simulink model "Tester_Controller_A"  (R2024b)
settings: Solver=VariableStepAuto  StartTime=0.0  StopTime=inf  RelTol=1e-3
values from neighbouring files (symbols this model uses):
  clegg = 0.55298    [Lookup_Tables_and_Initializer.m]
  D1 = 0.051209    [Lookup_Tables_and_Initializer.m]
  D2 = 0.050783    [Lookup_Tables_and_Initializer.m]
  E_table = E(V_range2,h_funct(Max_Terminal_V_factor),Sharpness_Const)    [Lookup_Tables.m]    (also in Lookup_Tables_and_Initializer.m)
  I1 = 1.3154    [Lookup_Tables_and_Initializer.m]
  I2 = 0.51307    [Lookup_Tables_and_Initializer.m]
  P1 = 2.4635    [Lookup_Tables_and_Initializer.m]
  P2 = 0.29756    [Lookup_Tables_and_Initializer.m]
  V_range2 = 0:0.01:1.44    [Lookup_Tables.m]    (also in Lookup_Tables_and_Initializer.m)
undefined symbols (not defined in the file or in its folder): DiscIntNeverNeededParam
libraries: simulink x3, slpidlib x3, eeGeneralControl x2, instrumentlib x2, dspstat3 x1, dspindex x1, realtime_pacer_lib x1, SignalEditorBlockLib x1
settings Model: Creator=errikos  LastModifiedBy=sh2323
settings SolverCC: AlgebraicLoopSolver=TrustRegion
settings DataIOCC: ReturnWorkspaceOutputs=off
settings DebuggingCC: UnconnectedInputMsg=warning  UnconnectedOutputMsg=warning  UnconnectedLineMsg=warning  ArithmeticOperatorsInVariantConditions=warning
settings ModelReferenceCC: EnableRefExpFcnMdlSchedulingChecks=on
settings SFSimCC: CustomCodeUndefinedFunction=UseInterfaceOnly
settings RTWCC: GPUComputeCapability=3.5  DLArmComputeVersion=19.05

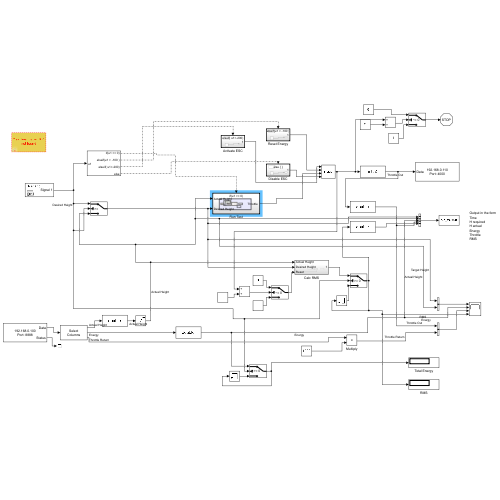
[thumbnail: Simulink's stored preview of the top-level diagram]
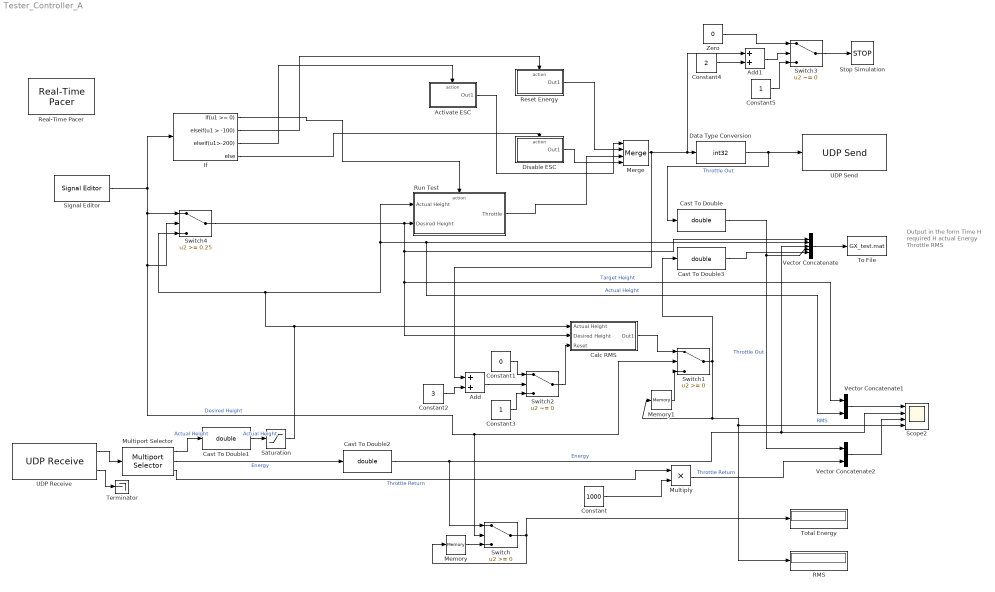
== system Tester_Controller_A ==
  note: Output in the form
      | Time
      | H required
      | H actual
      | Energy
      | Throttle
      | RMS
  Activate ESC : Subsystem  TreatAsAtomicUnit=on
  Add : Sum
  Add1 : Sum
  Calc RMS : Subsystem
  Cast To Double{,1..3} (4 alike) : DataTypeConversion  OutDataTypeStr=double  SaturateOnIntegerOverflow=off  RndMeth=Floor
  Constant : Constant  Value=1000
  Constant1 : Constant  Value=0
  Constant2 : Constant  Value=3
  Constant3 : Constant
  Constant4 : Constant  Value=2
  Constant5 : Constant
  Data Type Conversion : DataTypeConversion  OutDataTypeStr=int32  SaturateOnIntegerOverflow=off  RndMeth=Floor
  Disable ESC : Subsystem  TreatAsAtomicUnit=on
  If : If  IfExpression=u1 >= 0  ElseIfExpressions=u1 > -100 , u1>-200
  Memory : Memory
  Memory1 : Memory
  Merge : Merge  Inputs=4
  Multiply : Product
  Multiport Selector : dspindex/Multiport Selector  rowsOrCols=Columns  idxCellArray={ 1, 2,3}  idxErrMode=Clip and Warn
  RMS : Display
  Real-Time Pacer : realtime_pacer_lib/Real-Time Pacer  simTimePerRealTime=1
  Reset Energy : Subsystem  TreatAsAtomicUnit=on
  Run Test : Subsystem  TreatAsAtomicUnit=on
  Saturation : Saturate  UpperLimit=1.7  LowerLimit=0
  Scope2 : Scope  NumInputPorts=4
  Signal Editor : SignalEditorBlockLib/Signal Editor  FileName=/Users/errikoslevis/Downloads/Simulink Testing/samplemission.mat  ActiveScenario=Scenario  ActiveSignal=Signal 1  IsBus=off  OutputBusObjectStr=Bus: BusObject  SampleTime=0.05  ZeroCross=off  OutputAfterFinalValue=Setting to zero  Unit=inherit  PreserveSignalName=on  ApplySigPropsToAllScenarios=on  ApplySigPropsToAllSignals=off
  Stop Simulation : Stop
  Switch : Switch  SaturateOnIntegerOverflow=off  InputSameDT=off
  Switch1 : Switch  SaturateOnIntegerOverflow=off  InputSameDT=off
  Switch2 : Switch  Criteria=u2 ~= 0  SaturateOnIntegerOverflow=off  InputSameDT=off
  Switch3 : Switch  Criteria=u2 ~= 0  ZeroCross=off  SaturateOnIntegerOverflow=off  InputSameDT=off
  Switch4 : Switch  Threshold=0.25  SaturateOnIntegerOverflow=off  InputSameDT=off
  Terminator : Terminator
  To File : ToFile  Filename=GX_test.mat
  Total Energy : Display
  UDP Receive : instrumentlib/UDP Receive  LocalAddress=192.168.0.100  LocalPort=8888  EnablePortSharing=on  Host=192.168.0.110  Port=4000  GetLatestData=on  DataSize="[1  3]"  DataType=single  ASCIIFormatting=%f%f  Terminator=LF  CustomTerminator=10  ByteOrder=little-endian  EnableBlockingMode=off  Timeout=10  SampleTime=0.05  SimulateUsing=Interpreted execution
  UDP Send : instrumentlib/UDP Send  Host=192.168.0.110  Port=4000  LocalAddress=192.168.0.100  LocalPort=-1  EnablePortSharing=on  OutputDatagramPacketSize=4  ByteOrder=little-endian  EnableBlockingMode=on  SimulateUsing=Interpreted execution
  Vector Concatenate : Concatenate  NumInputs=5
  Vector Concatenate1 : Concatenate
  Vector Concatenate2 : Concatenate
  Zero : Constant  Value=0  OutDataTypeStr=Inherit: Inherit via back propagation
  wires:
  UDP Receive/1 -> Multiport Selector/1
  Multiport Selector/1 -> Cast To Double1/1  "Actual Height"
  Multiport Selector/2 -> Cast To Double2/1  "Energy"
  Run Test/1("Throttle ") -> Merge/3
  Data Type Conversion/1 -> Cast To Double/1, UDP Send/1  "Throttle Out"
  Multiport Selector/3 -> Multiply/1  "Throttle Return"
  Multiply/1 -> Vector Concatenate2/2  "Throttle Return"
  Constant/1 -> Multiply/2
  Signal Editor/1 -> Switch4/2, Switch1/2, Switch/2, Switch4/1, If/1  "Desired Height"
  Merge/1 -> Add/1, Add1/1, Data Type Conversion/1
  Vector Concatenate/1 -> To File/1
  If/1 -> Run Test/Action
  If/2 -> Reset Energy/Action
  If/3 -> Activate ESC/Action
  If/4 -> Disable ESC/Action
  Activate ESC/1(Out1) -> Merge/1
  Disable ESC/1(Out1) -> Merge/4
  Switch/1 -> Memory/1, Total Energy/1
  Cast To Double/1 -> Vector Concatenate2/1, Vector Concatenate/4  "Throttle Out"
  Saturation/1 -> Switch4/3, Run Test/1(Actual Height), Vector Concatenate1/2, Vector Concatenate/2, Calc RMS/1(Actual Height)  "Actual Height"
  Cast To Double2/1 -> Switch/1, Scope2/2, Vector Concatenate/3  "Energy"
  Cast To Double3/1 -> Vector Concatenate/5
  Memory/1 -> Switch/3
  Switch1/1 -> RMS/1, Scope2/4, Memory1/1, Cast To Double3/1  "RMS"
  Memory1/1 -> Switch1/3
  Calc RMS/1(Out1) -> Switch1/1
  Switch2/1 -> Calc RMS/3(Reset)
  Constant1/1 -> Switch2/1
  Constant2/1 -> Add/2
  Add/1 -> Switch2/2
  Constant3/1 -> Switch2/3
  Reset Energy/1(Out1) -> Merge/2
  Switch3/1 -> Stop Simulation/1
  Zero/1 -> Switch3/1
  Add1/1 -> Switch3/2
  Constant4/1 -> Add1/2
  Constant5/1 -> Switch3/3
  Vector Concatenate2/1 -> Scope2/3
  Vector Concatenate1/1 -> Scope2/1
  Switch4/1 -> Vector Concatenate/1, Vector Concatenate1/1, Calc RMS/2(Desired Height), Run Test/2(Desired Height)  "Target Height"
  Cast To Double1/1 -> Saturation/1  "Actual Height"
  UDP Receive/2 -> Terminator/1

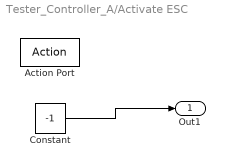
== system Tester_Controller_A/Activate ESC ==
  Action Port : ActionPort  ActionPortLabel=elseif( u1>-200)
  Constant : Constant  Value=-1  SampleTime=0.05
  Out1 : Outport  VectorParamsAs1DForOutWhenUnconnected=off
  wires:
  Constant/1 -> Out1/1

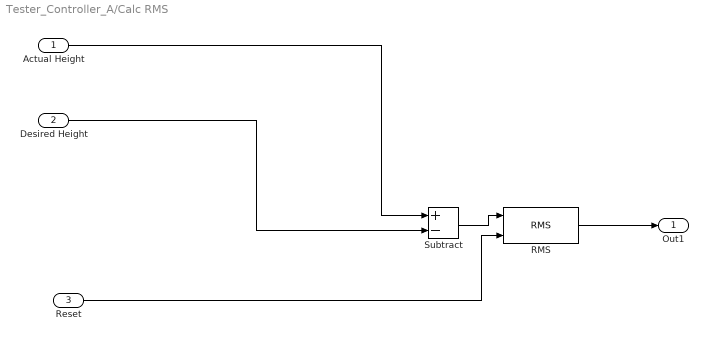
== system Tester_Controller_A/Calc RMS ==
  Actual Height : Inport
  Desired Height : Inport  Port=2
  Reset : Inport  Port=3
  RMS : dspstat3/RMS  run=on  directionMode=Each column  dimension=1  reset_popup=Non-zero sample
  Subtract : Sum  Inputs=+-
  Out1 : Outport  VectorParamsAs1DForOutWhenUnconnected=off
  wires:
  Desired Height/1 -> Subtract/2
  Actual Height/1 -> Subtract/1
  RMS/1 -> Out1/1
  Subtract/1 -> RMS/1
  Reset/1 -> RMS/2

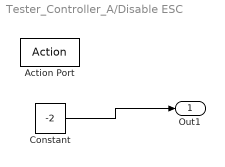
== system Tester_Controller_A/Disable ESC ==
  Action Port : ActionPort  ActionPortLabel=else
  Constant : Constant  Value=-2  SampleTime=0.05
  Out1 : Outport  VectorParamsAs1DForOutWhenUnconnected=off
  wires:
  Constant/1 -> Out1/1

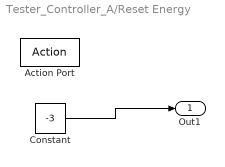
== system Tester_Controller_A/Reset Energy ==
  Action Port : ActionPort  ActionPortLabel=elseif(u1 > -100 )
  Constant : Constant  Value=-3  SampleTime=0.05
  Out1 : Outport  VectorParamsAs1DForOutWhenUnconnected=off
  wires:
  Constant/1 -> Out1/1

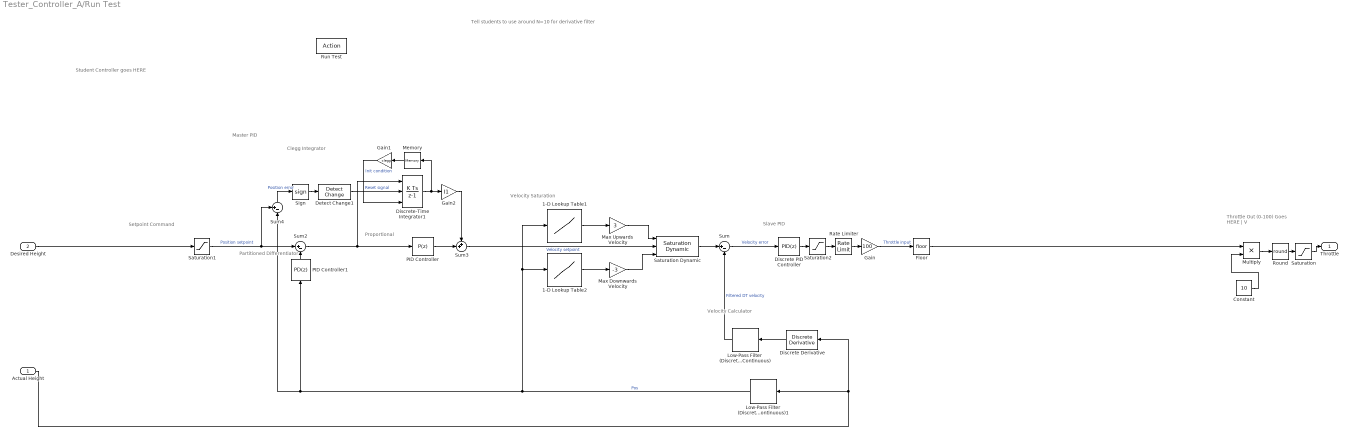
== system Tester_Controller_A/Run Test ==
  note: Tell students to use around N=10 for derivative filter
  note: Throttle Out (0-100)
      | Goes HERE
      |            |
      | 	   V
  note: Student Controller goes HERE
  note: Velocity Calculator
  note: Setpoint Command
  note: Partitioned
      | Differentiator
  note: Proportional
  note: Clegg Integrator
  note: Master
      | PID
  note: Velocity Saturation
  note: Slave PID
  Actual Height : Inport
  Desired Height : Inport  Port=2
  Run Test : ActionPort  ActionPortLabel=if(u1 >= 0)
  1-D Lookup Table1 : Lookup_n-D  NumberOfTableDimensions=1  BreakpointsForDimension1=V_range2  Table=flip(E_table)  InterpMethod=Nearest  InternalRulePriority=Speed  RndMeth=Simplest
  1-D Lookup Table2 : Lookup_n-D  NumberOfTableDimensions=1  BreakpointsForDimension1=V_range2  Table=E_table  InterpMethod=Nearest  InternalRulePriority=Speed  RndMeth=Simplest
  Constant : Constant  Value=10
  Detect Change1 : simulink/Logic and Bit Operations/Detect Change  vinit=0  OutDataTypeStr=boolean
  Discrete Derivative : simulink/Discrete/Discrete Derivative  gainval=1.0  ICPrevScaledInput=0.0  OutMin=[]  OutMax=[]  OutDataType=fixdt(1, 16)  OutScaling=2^-10  DoSatur=off
  Discrete PID Controller : slpidlib/PID Controller  Controller=PID  Form=Parallel  TimeDomain=Discrete-time  UseExternalTs=off  SampleTime=-1  IntegratorMethod=Forward Euler  FilterMethod=Forward Euler  ControllerParametersSource=internal  P=P2  I=I2  UseKiTs=off  D=D2  UseExternalDerivativeSource=off  N=10  UseFilter=on  TunerSelectOption=Transfer Function Based (PID Tuner App)  InitialConditionSource=internal  InitialConditionForIntegrator=0  InitialConditionForFilter=0  DifferentiatorICPrevScaledInput=0  ExternalReset=none  TrackingMode=off  Kt=1  LimitOutput=on  SatLimitsSource=internal  UpperSaturationLimit=1  LowerSaturationLimit=0  LinearizeAsGain=off  AntiWindupMode=none  Kb=1  LimitIntegrator=off  UpperIntegratorSaturationLimit=inf  LowerIntegratorSaturationLimit=-inf  POutMin=[]  POutMax=[]  IOutMin=[]  IOutMax=[]  DOutMin=[]  DOutMax=[]  NOutMin=[]  NOutMax=[]  SumOutMin=[]  SumOutMax=[]  SaturationOutMin=[]  SaturationOutMax=[]  PParamMin=[]  PParamMax=[]  IParamMin=[]  IParamMax=[]  DParamMin=[]  DParamMax=[]  NParamMin=[]  NParamMax=[]  KbParamMin=[]  KbParamMax=[]  KtParamMin=[]  KtParamMax=[]  KbOutMin=[]  KbOutMax=[]  KtOutMin=[]  KtOutMax=[]  IntegratorOutMin=[]  IntegratorOutMax=[]  FilterOutMin=[]  FilterOutMax=[]  SumI1OutMin=[]  SumI1OutMax=[]  SumI2OutMin=[]  SumI2OutMax=[]  SumI3OutMin=[]  SumI3OutMax=[]  SumI4OutMin=[]  SumI4OutMax=[]  SumDOutMin=[]  SumDOutMax=[]  DifferentiatorOutMin=[]  DifferentiatorOutMax=[]  FilterDiffOutCoefMin=[]  FilterDiffOutCoefMax=[]  ReciprocalOutMin=[]  ReciprocalOutMax=[]  SumDenOutMin=[]  SumDenOutMax=[]  SumNumOutMin=[]  SumNumOutMax=[]  DivideOutMin=[]  DivideOutMax=[]  UdiffTsProdOutMin=[]  UdiffTsProdOutMax=[]  NTsProdOutMin=[]  NTsProdOutMax=[]  UintegralTsProdOutMin=[]  UintegralTsProdOutMax=[]  UngainTsProdOutMin=[]  UngainTsProdOutMax=[]  ClampingZeroOutDataTypeStr=Inherit: Inherit via back propagation  ClampingZeroOutMin=[]  ClampingZeroOutMax=[]  FilterDenConstantOutDataTypeStr=Inherit: Inherit via back propagation  FilterDenConstantOutMin=[]  FilterDenConstantOutMax=[]  PCopyOutDataTypeStr=Inherit: Inherit via back propagation  PCopyOutMin=[]  PCopyOutMax=[]  NCopyOutDataTypeStr=Inherit: Inherit via back propagation  NCopyOutMin=[]  NCopyOutMax=[]  IntegratorContinuousStateAttributes=''  IntegratorStateMustResolveToSignalObject=off  IntegratorRTWStateStorageClass=Auto  FilterContinuousStateAttributes=''  FilterStateMustResolveToSignalObject=off  FilterRTWStateStorageClass=Auto  ParallelPVariant=InternalParameters  IdealPVariant=Disabled  IVariant=InternalParameters  DVariant=InternalParameters  IntegratorVariant=Discrete  SatVariant=Enabled  AWVariant=Passthrough  PCopyVariant=Disabled  TRVariant=Disabled  FdbkBlocksVariant=Forward  IdealPFdbkVariant=Disabled  SatFdbkVariant=Disabled  DerivativeFilterVariant=ForwardEulerFilter  NVariant=InternalParameters  NCopyVariant=Disabled  FilterICVariant=InternalICsFilter  IntegratorICVariant=InternalICs  ExternalResetVariant=Disabled  TRSumVariant=Passthrough  SumFdbkVariant=Disabled  SumVariant=Sum_PID  TsampFilterVariant=InternalTs  TsampNgainVariant=Passthrough  TsampIntegralVariant=Disabled_SignalSpec  ExternalSaturationOutDataTypeStr=Inherit: Same as second input  DerivativeSourceVariant=ErrorSignal  PreIntVariant=InternalPreInt
      settings: LibrarySourceBlock=simulink/Discrete/Discrete PID Controller
  Discrete-Time Integrator1 : DiscreteIntegrator  ExternalReset=level  InitialConditionSource=external  SampleTime=-1  ICPrevOutput=DiscIntNeverNeededParam  ICPrevScaledInput=DiscIntNeverNeededParam
  Floor : Rounding
  Gain : Gain  Gain=100
  Gain1 : Gain  Gain=clegg
  Gain2 : Gain  Gain=I1
  Low-Pass Filter (Discrete or Continuous) : eeGeneralControl/Low-Pass Filter (Discrete or Continuous)  K=1  T=0.075  B=inf  A=-inf  init_option=Inherited from block input  x0=0  Ts=-1
  Low-Pass Filter (Discrete or Continuous)1 : eeGeneralControl/Low-Pass Filter (Discrete or Continuous)  K=1  T=0.075  B=inf  A=-inf  init_option=Inherited from block input  x0=0  Ts=-1
  Max Downwards Velocity : Gain  Gain=-3
  Max Upwards Velocity : Gain  Gain=3
  Memory : Memory
  Multiply : Product
  PID Controller : slpidlib/PID Controller  Controller=P  Form=Parallel  TimeDomain=Discrete-time  UseExternalTs=off  SampleTime=-1  IntegratorMethod=Forward Euler  FilterMethod=Forward Euler  ControllerParametersSource=internal  P=P1  I=4  UseKiTs=off  D=0  UseExternalDerivativeSource=off  N=10  UseFilter=on  TunerSelectOption=Transfer Function Based (PID Tuner App)  InitialConditionSource=internal  InitialConditionForIntegrator=0  InitialConditionForFilter=0  DifferentiatorICPrevScaledInput=0  ExternalReset=none  TrackingMode=off  Kt=1  LimitOutput=off  SatLimitsSource=internal  UpperSaturationLimit=inf  LowerSaturationLimit=-inf  LinearizeAsGain=on  AntiWindupMode=none  Kb=1  LimitIntegrator=off  UpperIntegratorSaturationLimit=inf  LowerIntegratorSaturationLimit=-inf  POutMin=[]  POutMax=[]  IOutMin=[]  IOutMax=[]  DOutMin=[]  DOutMax=[]  NOutMin=[]  NOutMax=[]  SumOutMin=[]  SumOutMax=[]  SaturationOutMin=[]  SaturationOutMax=[]  PParamMin=[]  PParamMax=[]  IParamMin=[]  IParamMax=[]  DParamMin=[]  DParamMax=[]  NParamMin=[]  NParamMax=[]  KbParamMin=[]  KbParamMax=[]  KtParamMin=[]  KtParamMax=[]  KbOutMin=[]  KbOutMax=[]  KtOutMin=[]  KtOutMax=[]  IntegratorOutMin=[]  IntegratorOutMax=[]  FilterOutMin=[]  FilterOutMax=[]  SumI1OutMin=[]  SumI1OutMax=[]  SumI2OutMin=[]  SumI2OutMax=[]  SumI3OutMin=[]  SumI3OutMax=[]  SumI4OutMin=[]  SumI4OutMax=[]  SumDOutMin=[]  SumDOutMax=[]  DifferentiatorOutMin=[]  DifferentiatorOutMax=[]  FilterDiffOutCoefMin=[]  FilterDiffOutCoefMax=[]  ReciprocalOutMin=[]  ReciprocalOutMax=[]  SumDenOutMin=[]  SumDenOutMax=[]  SumNumOutMin=[]  SumNumOutMax=[]  DivideOutMin=[]  DivideOutMax=[]  UdiffTsProdOutMin=[]  UdiffTsProdOutMax=[]  NTsProdOutMin=[]  NTsProdOutMax=[]  UintegralTsProdOutMin=[]  UintegralTsProdOutMax=[]  UngainTsProdOutMin=[]  UngainTsProdOutMax=[]  ClampingZeroOutDataTypeStr=Inherit: Inherit via back propagation  ClampingZeroOutMin=[]  ClampingZeroOutMax=[]  FilterDenConstantOutDataTypeStr=Inherit: Inherit via back propagation  FilterDenConstantOutMin=[]  FilterDenConstantOutMax=[]  PCopyOutDataTypeStr=Inherit: Inherit via back propagation  PCopyOutMin=[]  PCopyOutMax=[]  NCopyOutDataTypeStr=Inherit: Inherit via back propagation  NCopyOutMin=[]  NCopyOutMax=[]  IntegratorContinuousStateAttributes=''  IntegratorStateMustResolveToSignalObject=off  IntegratorRTWStateStorageClass=Auto  FilterContinuousStateAttributes=''  FilterStateMustResolveToSignalObject=off  FilterRTWStateStorageClass=Auto  ParallelPVariant=InternalParameters  IdealPVariant=Disabled  IVariant=Disabled  DVariant=Disabled  IntegratorVariant=Disabled  SatVariant=Disabled  AWVariant=Disabled  PCopyVariant=Disabled  TRVariant=Disabled  FdbkBlocksVariant=Forward  IdealPFdbkVariant=Disabled  SatFdbkVariant=Disabled  DerivativeFilterVariant=Disabled  NVariant=Disabled  NCopyVariant=Disabled_SignalSpec  FilterICVariant=Disabled  IntegratorICVariant=Disabled  ExternalResetVariant=Disabled  TRSumVariant=Passthrough  SumFdbkVariant=Disabled  SumVariant=Passthrough_P  TsampFilterVariant=InternalTs  TsampNgainVariant=Passthrough  TsampIntegralVariant=Disabled_SignalSpec  ExternalSaturationOutDataTypeStr=Inherit: Same as second input  DerivativeSourceVariant=Disabled  PreIntVariant=InternalPreInt
  PID Controller1 : slpidlib/PID Controller  Controller=PD  Form=Parallel  TimeDomain=Discrete-time  UseExternalTs=off  SampleTime=-1  IntegratorMethod=Forward Euler  FilterMethod=Forward Euler  ControllerParametersSource=internal  P=1  I=1  UseKiTs=off  D=D1/P1  UseExternalDerivativeSource=off  N=10  UseFilter=on  TunerSelectOption=Transfer Function Based (PID Tuner App)  InitialConditionSource=internal  InitialConditionForIntegrator=0  InitialConditionForFilter=0  DifferentiatorICPrevScaledInput=0  ExternalReset=none  TrackingMode=off  Kt=1  LimitOutput=off  SatLimitsSource=internal  UpperSaturationLimit=inf  LowerSaturationLimit=-inf  LinearizeAsGain=on  AntiWindupMode=none  Kb=1  LimitIntegrator=off  UpperIntegratorSaturationLimit=inf  LowerIntegratorSaturationLimit=-inf  POutMin=[]  POutMax=[]  IOutMin=[]  IOutMax=[]  DOutMin=[]  DOutMax=[]  NOutMin=[]  NOutMax=[]  SumOutMin=[]  SumOutMax=[]  SaturationOutMin=[]  SaturationOutMax=[]  PParamMin=[]  PParamMax=[]  IParamMin=[]  IParamMax=[]  DParamMin=[]  DParamMax=[]  NParamMin=[]  NParamMax=[]  KbParamMin=[]  KbParamMax=[]  KtParamMin=[]  KtParamMax=[]  KbOutMin=[]  KbOutMax=[]  KtOutMin=[]  KtOutMax=[]  IntegratorOutMin=[]  IntegratorOutMax=[]  FilterOutMin=[]  FilterOutMax=[]  SumI1OutMin=[]  SumI1OutMax=[]  SumI2OutMin=[]  SumI2OutMax=[]  SumI3OutMin=[]  SumI3OutMax=[]  SumI4OutMin=[]  SumI4OutMax=[]  SumDOutMin=[]  SumDOutMax=[]  DifferentiatorOutMin=[]  DifferentiatorOutMax=[]  FilterDiffOutCoefMin=[]  FilterDiffOutCoefMax=[]  ReciprocalOutMin=[]  ReciprocalOutMax=[]  SumDenOutMin=[]  SumDenOutMax=[]  SumNumOutMin=[]  SumNumOutMax=[]  DivideOutMin=[]  DivideOutMax=[]  UdiffTsProdOutMin=[]  UdiffTsProdOutMax=[]  NTsProdOutMin=[]  NTsProdOutMax=[]  UintegralTsProdOutMin=[]  UintegralTsProdOutMax=[]  UngainTsProdOutMin=[]  UngainTsProdOutMax=[]  ClampingZeroOutDataTypeStr=Inherit: Inherit via back propagation  ClampingZeroOutMin=[]  ClampingZeroOutMax=[]  FilterDenConstantOutDataTypeStr=Inherit: Inherit via back propagation  FilterDenConstantOutMin=[]  FilterDenConstantOutMax=[]  PCopyOutDataTypeStr=Inherit: Inherit via back propagation  PCopyOutMin=[]  PCopyOutMax=[]  NCopyOutDataTypeStr=Inherit: Inherit via back propagation  NCopyOutMin=[]  NCopyOutMax=[]  IntegratorContinuousStateAttributes=''  IntegratorStateMustResolveToSignalObject=off  IntegratorRTWStateStorageClass=Auto  FilterContinuousStateAttributes=''  FilterStateMustResolveToSignalObject=off  FilterRTWStateStorageClass=Auto  ParallelPVariant=InternalParameters  IdealPVariant=Disabled  IVariant=Disabled  DVariant=InternalParameters  IntegratorVariant=Disabled  SatVariant=Disabled  AWVariant=Disabled  PCopyVariant=Disabled  TRVariant=Disabled  FdbkBlocksVariant=Forward  IdealPFdbkVariant=Disabled  SatFdbkVariant=Disabled  DerivativeFilterVariant=ForwardEulerFilter  NVariant=InternalParameters  NCopyVariant=Disabled  FilterICVariant=InternalICsFilter  IntegratorICVariant=Disabled  ExternalResetVariant=Disabled  TRSumVariant=Passthrough  SumFdbkVariant=Disabled  SumVariant=Sum_PD  TsampFilterVariant=InternalTs  TsampNgainVariant=Passthrough  TsampIntegralVariant=Disabled_SignalSpec  ExternalSaturationOutDataTypeStr=Inherit: Same as second input  DerivativeSourceVariant=ErrorSignal  PreIntVariant=InternalPreInt
  Rate Limiter : RateLimiter  RisingSlewLimit=8  FallingSlewLimit=-8  SampleTimeMode=inherited
  Round : Rounding  Operator=round
  Saturation : Saturate  UpperLimit=1000  LowerLimit=0
  Saturation Dynamic : simulink/Discontinuities/Saturation Dynamic  OutMin=[]  OutMax=[]  OutDataTypeStr=Inherit: Same as second input  OutDataType=fixdt(1, 16)  OutScaling=2^-10  DoSatur=off
  Saturation1 : Saturate  UpperLimit=1.44  LowerLimit=0
  Saturation2 : Saturate  UpperLimit=0.9  LowerLimit=0
  Sign : Signum
  Sum : Sum  Inputs=|+-
  Sum2 : Sum  Inputs=|+-
  Sum3 : Sum  Inputs=++|
  Sum4 : Sum  Inputs=+-|
  "Throttle " : Outport  VectorParamsAs1DForOutWhenUnconnected=off
  wires:
  Saturation/1 -> "Throttle "/1
  Constant/1 -> Multiply/2
  Multiply/1 -> Round/1
  Round/1 -> Saturation/1
  Floor/1 -> Multiply/1
  Gain/1 -> Floor/1  "Throttle input"
  Memory/1 -> Gain1/1
  Sum3/1 -> Saturation Dynamic/2  "Velocity setpoint"
  Max Upwards Velocity/1 -> Saturation Dynamic/1
  Sum/1 -> Discrete PID Controller/1  "Velocity error"
  Discrete PID Controller/1 -> Saturation2/1
  Sign/1 -> Detect Change1/1
  Detect Change1/1 -> Discrete-Time Integrator1/2  "Reset signal"
  Saturation1/1 -> Sum2/1, Sum4/1  "Position setpoint"
  1-D Lookup Table2/1 -> Max Downwards Velocity/1
  Rate Limiter/1 -> Gain/1
  Discrete-Time Integrator1/1 -> Gain2/1, Memory/1
  Max Downwards Velocity/1 -> Saturation Dynamic/3
  Gain1/1 -> Discrete-Time Integrator1/3  "Init condition"
  Low-Pass Filter (Discrete or Continuous)1/1 -> 1-D Lookup Table1/1, 1-D Lookup Table2/1, PID Controller1/1, Sum4/2  "Pos"
  Gain2/1 -> Sum3/1
  PID Controller/1 -> Sum3/2
  Sum4/1 -> Sign/1  "Position error"
  1-D Lookup Table1/1 -> Max Upwards Velocity/1
  Saturation2/1 -> Rate Limiter/1
  PID Controller1/1 -> Sum2/2
  Low-Pass Filter (Discrete or Continuous)/1 -> Sum/2  "Filtered DT velocity"
  Saturation Dynamic/1 -> Sum/1
  Sum2/1 -> PID Controller/1, Discrete-Time Integrator1/1
  Discrete Derivative/1 -> Low-Pass Filter (Discrete or Continuous)/1
  Desired Height/1 -> Saturation1/1
  Actual Height/1 -> Discrete Derivative/1, Low-Pass Filter (Discrete or Continuous)1/1
